simulink subsystem "refrence_setter"  (R2022b)
settings: Solver=VariableStepAuto  StartTime=0.0  StopTime=10.0  RelTol=1e-3
model mask{time_stamps=[0 5 10], actuation=[0 5 10]}
  mask prompts: time_stamps "Time stamps"
settings Model: DefaultTestHarness=refrence_setter_Harness1  Creator=laula  LastModifiedBy=laula

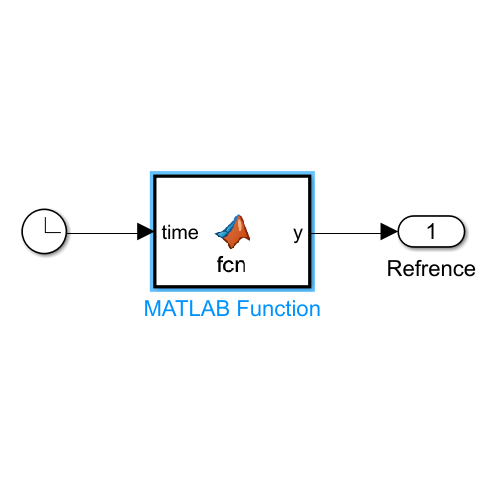
[thumbnail: Simulink's stored preview of the top-level diagram]
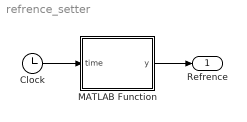
== system refrence_setter ==
  Clock : Clock
  MATLAB Function : MATLAB Function  TreatAsAtomicUnit=on
  Refrence : Outport
  wires:
  Clock/1 -> MATLAB Function/1(time)
  MATLAB Function/1(y) -> Refrence/1

== matlab function refrence_setter/MATLAB Function ==
  data: time input; y output; time_stamps parameter; actuation parameter
function y = fcn(time, time_stamps, actuation)


greater_than = time > time_stamps - 0.01;

index = sum(greater_than);

if(index > length(time_stamps))
    index = index - 1
end

y = actuation(index);
